simulink library "Feeder2_lib"  (Simulink 8.1)
settings: Solver=ode45  StartTime=0.0  StopTime=10.0  RelTol=1e-3
undefined symbols (not defined in the file): Left, Ts, type, V
libraries: breaker_lib x20, cables_lib x14, transformer_lib x12, Load_lib x8, ssn_lib x7, powerlib x4, fault_lib x2, rtlab x2
settings Model: Creator=re25624  LastModifiedBy=RE25624

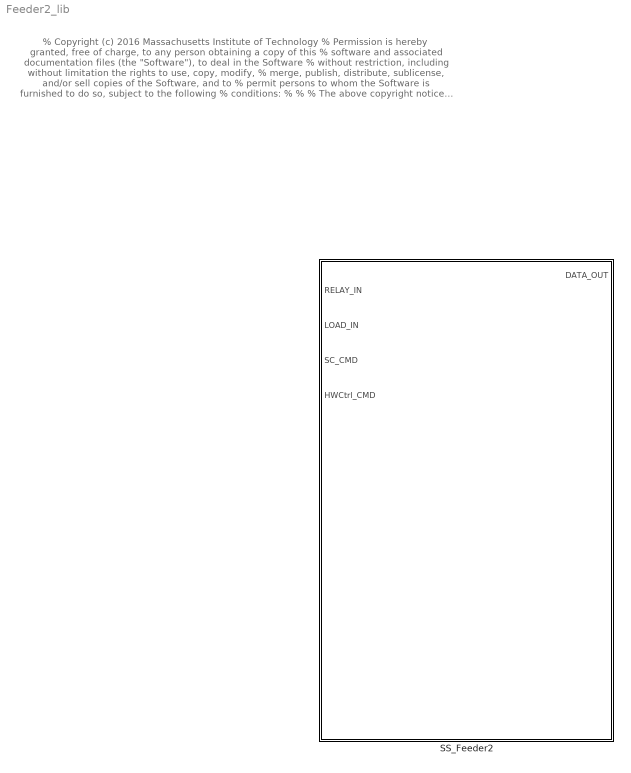
== system Feeder2_lib ==
  note: % Copyright (c) 2016 Massachusetts Institute of Technology
      | % Permission is hereby granted, free of charge, to any person obtaining a copy of this
      | % software and associated documentation files (the "Software"), to deal in the Software
      | % without restriction, including without limitation the rights to use, copy, modify,
      | % merge, publish, distribute, sublicense, and/or sell copies of the Software, and to
      | % permit persons to whom the Software is furnished to do so, subject to the following
      | % conditions:
      | %
      | %
      | % The above copyright notice and this permission notice shall be included in
      | % all copies or substantial portions of the Software.
      | %
      | % THE SOFTWARE IS PROVIDED "AS IS", WITHOUT WARRANTY OF ANY KIND, EXPRESS OR IMPLIED,
      | % INCLUDING BUT NOT LIMITED TO THE WARRANTIES OF MERCHANTABILITY, FITNESS FOR A
      | % PARTICULAR PURPOSE AND NONINFRINGEMENT. IN NO EVENT SHALL THE AUTHORS OR COPYRIGHT
      | % HOLDERS BE LIABLE FOR ANY CLAIM, DAMAGES OR OTHER LIABILITY, WHETHER IN AN ACTION
      | % OF CONTRACT, TORT OR OTHERWISE, ARISING FROM, OUT OF OR IN CONNECTION WITH THE
      | % SOFTWARE OR THE USE OR OTHER DEALINGS IN THE SOFTWARE.
      | %
      | %
      | %%
  SS_Feeder2 : Subsystem

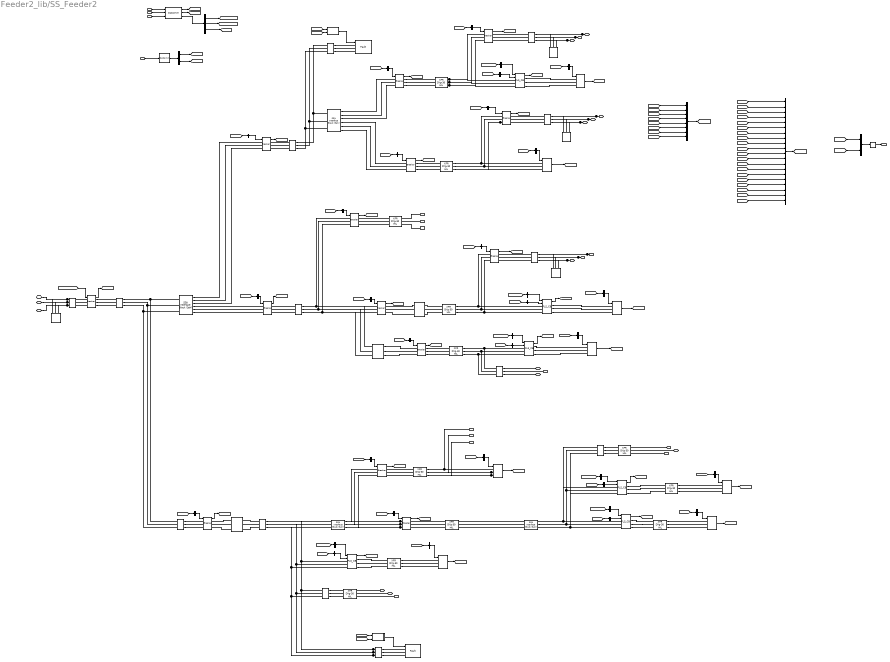
== system Feeder2_lib/SS_Feeder2 ==
  note: BESS SYSTEM
  note: % Copyright (c) 2016 Massachusetts Institute of Technology
      | % Permission is hereby granted, free of charge, to any person obtaining a copy of this
      | % software and associated documentation files (the "Software"), to deal in the Software
      | % without restriction, including without limitation the rights to use, copy, modify,
      | % merge, publish, distribute, sublicense, and/or sell copies of the Software, and to
      | % permit persons to whom the Software is furnished to do so, subject to the following
      | % conditions:
      | %
      | %
      | % The above copyright notice and this permission notice shall be included in
      | % all copies or substantial portions of the Software.
      | %
      | % THE SOFTWARE IS PROVIDED "AS IS", WITHOUT WARRANTY OF ANY KIND, EXPRESS OR IMPLIED,
      | % INCLUDING BUT NOT LIMITED TO THE WARRANTIES OF MERCHANTABILITY, FITNESS FOR A
      | % PARTICULAR PURPOSE AND NONINFRINGEMENT. IN NO EVENT SHALL THE AUTHORS OR COPYRIGHT
      | % HOLDERS BE LIABLE FOR ANY CLAIM, DAMAGES OR OTHER LIABILITY, WHETHER IN AN ACTION
      | % OF CONTRACT, TORT OR OTHERWISE, ARISING FROM, OUT OF OR IN CONNECTION WITH THE
      | % SOFTWARE OR THE USE OR OTHER DEALINGS IN THE SOFTWARE.
      | %
      | %
      | %%
  note: connect to F1
  note: PV SYSTEM
  note: connect to F3
  note: connect to F3
  note: connect to F3
  note: connect to F1
  note: connect to F1
  RELAY_IN : Inport
  LOAD_IN : Inport  Port=2
  SC_CMD : Inport  Port=3
  HWCtrl_CMD : Inport  Port=4
  1000 kVA1 : transformer_lib/XFR DYg-30 HIL  Rating=1000  Vp=13800  Vs=480  Z=4.56  XR=4.49
  1000 kVA2 : transformer_lib/XFR DYg-30 HIL  Rating=1000  Vp=4160  Vs=480  Z=5.56  XR=5.49
  1500 kVA : transformer_lib/XFR DYg-30 HIL  Rating=1500  Vp=4160  Vs=480  Z=5.56  XR=5.51
  2000 kVA2 : transformer_lib/XFR DYg-30 HIL  Rating=2000  Vp=13800  Vs=480  Z=3  XR=5.7
  2000 kVA3 : transformer_lib/XFR DYg-30 HIL  Rating=2000  Vp=13800  Vs=480  Z=3  XR=5.7
  2500 kVA : transformer_lib/XFR DYg-30 HIL  Rating=2500  Vp=13800  Vs=480  Z=5.56  XR=5.52
  2500 kVA1 : transformer_lib/XFR DYg-30 HIL  Rating=2500  Vp=13800  Vs=480  Z=3.56  XR=5.52
  3750 kVA : transformer_lib/XFR DYg-30 HIL  Rating=3750  Vp=13800  Vs=4160  Z=4.75  XR=11.4
  4/0AWG-Mutual : cables_lib/4//0AWG-Mutual  length=10  par_sets=1  ratio=3
  448 kvar inductor at 13.8kV  to cancel kvar produced by the stublines1 : powerlib/Elements/Three-Phase Parallel RLC Load  LConnTagsString=A|B|C  Configuration=Y (grounded)  NominalVoltage=13800  NominalFrequency=60  ActivePower=0  InductivePower=448e3  CapacitivePower=0  Measurements=None  LoadType=constant Z
  500 kVA : transformer_lib/XFR DYg-30 HIL  Rating=500  Vp=13800  Vs=208  Z=5  XR=4.9
  5000 kVA : transformer_lib/XFR DYg-30 HIL  Rating=5000  Vp=13800  Vs=480  Z=3  XR=5.44
  500kcmil-Mutual2 : cables_lib/500kcmil-Mutual  length=10  par_sets=1  ratio=3
  500kcmil-Mutual4 : cables_lib/500kcmil-Mutual  length=10  par_sets=1  ratio=3
  500kcmil-Mutual5 : cables_lib/500kcmil-Mutual  length=1000  par_sets=1  ratio=3
  500kcmil-Mutual8 : cables_lib/500kcmil-Mutual  length=100  par_sets=1  ratio=3
  500kcmil-Mutual9 : cables_lib/500kcmil-Mutual  length=10  par_sets=1  ratio=3
  6 kvar inductor at 480V  to cancel kvar produced by the stublines1 : powerlib/Elements/Three-Phase Parallel RLC Load  LConnTagsString=A|B|C  Configuration=Y (grounded)  NominalVoltage=480  NominalFrequency=60  ActivePower=0  InductivePower=6e3  CapacitivePower=0  Measurements=None  LoadType=constant Z
  6 kvar inductor at 480V  to cancel kvar produced by the stublines2 : powerlib/Elements/Three-Phase Parallel RLC Load  LConnTagsString=A|B|C  Configuration=Y (grounded)  NominalVoltage=480  NominalFrequency=60  ActivePower=0  InductivePower=6e3  CapacitivePower=0  Measurements=None  LoadType=constant Z
  6 kvar inductor at 480V  to cancel kvar produced by the stublines3 : powerlib/Elements/Three-Phase Parallel RLC Load  LConnTagsString=A|B|C  Configuration=Y (grounded)  NominalVoltage=480  NominalFrequency=60  ActivePower=0  InductivePower=6e3  CapacitivePower=0  Measurements=None  LoadType=constant Z
  Bus Creator2 : BusCreator  Inputs=2
  Bus Creator3 : BusCreator  Inputs=8
  Bus Creator5 : BusCreator  Inputs=20
  Bus Selector1 : BusSelector  OutputSignals=F2_CB_4
  Bus Selector10 : BusSelector  OutputSignals=I4
  Bus Selector11 : BusSelector  OutputSignals=F2_CB_11
  Bus Selector12 : BusSelector  OutputSignals=F2_CB_15
  Bus Selector13 : BusSelector  OutputSignals=F2_CB_3
  Bus Selector14 : BusSelector  OutputSignals=F2_CB_14
  Bus Selector15 : BusSelector  OutputSignals=F2_CB_17
  Bus Selector16 : BusSelector  OutputSignals=F2_CB_16
  Bus Selector17 : BusSelector  OutputSignals=F2_CB_13
  Bus Selector18 : BusSelector  OutputSignals=F2_CB_10
  Bus Selector19 : BusSelector  OutputSignals=F2_CB_9
  Bus Selector2 : BusSelector  OutputSignals=F2_CB_2
  Bus Selector20 : BusSelector  OutputSignals=F2_CB_12
  Bus Selector21 : BusSelector  OutputSignals=F2_CB_5
  Bus Selector22 : BusSelector  OutputSignals=F2_CB_7
  Bus Selector23 : BusSelector  OutputSignals=F2_CB_8
  Bus Selector24 : BusSelector  OutputSignals=F2_CB_6
  Bus Selector25 : BusSelector  OutputSignals=F2_CB_1
  Bus Selector26 : BusSelector  OutputSignals=F2_CB_18
  Bus Selector27 : BusSelector  OutputSignals=F2_CB_19
  Bus Selector28 : BusSelector  OutputSignals=fault_cmd,GridStatusCtrl.Grid_F2.Logic_trip
  Bus Selector29 : BusSelector  OutputSignals=HWCtrl.SEL751_LogicTrip.F2.Logic_trip,HWCtrl.SEL2440_FLS,TestSeq
  Bus Selector3 : BusSelector  OutputSignals=P5
  Bus Selector30 : BusSelector  OutputSignals=CB218
  Bus Selector31 : BusSelector  OutputSignals=CB212
  Bus Selector32 : BusSelector  OutputSignals=CB219
  Bus Selector33 : BusSelector  OutputSignals=CB206
  Bus Selector34 : BusSelector  OutputSignals=CB208
  Bus Selector35 : BusSelector  OutputSignals=CB204
  Bus Selector4 : BusSelector  OutputSignals=C4
  Bus Selector5 : BusSelector  OutputSignals=I5
  Bus Selector6 : BusSelector  OutputSignals=P2
  Bus Selector7 : BusSelector  OutputSignals=C3
  Bus Selector8 : BusSelector  OutputSignals=P3
  Bus Selector9 : BusSelector  OutputSignals=I3
  C{1..2,204..206} (5 alike) : cables_lib/500kcmil-Mutual  length=10  par_sets=1  ratio=3
  C201 : cables_lib/4//0AWG-Mutual  length=5500  par_sets=1  ratio=3
  C202 : cables_lib/500kcmil-Mutual  length=2000  par_sets=1  ratio=3
  C203 : cables_lib/500kcmil-Mutual  length=3000  par_sets=1  ratio=3
  Critical_3 : Load_lib/Dynamic_Load  V=480  kVA=1000  PF=0.9  Ts=Ts
  Critical_4 : Load_lib/Dynamic_Load  V=480  kVA=1000  PF=0.9  Ts=Ts
  F2_CB_{1..3,5,7,9..11,13..17} (13 alike) : breaker_lib/Breaker  Ts=Ts  mech_delay=cb_mech_delay
  F2_CB_{4,6,8,12,18..19} (6 alike) : breaker_lib/FLS_CB  Ts=Ts  mech_delay=cb_mech_delay
  F2_PCC : breaker_lib/Breaker  Ts=Ts  mech_delay=cb_mech_delay
  Fault_1 : fault_lib/Fault  FaultResistance=0.1  GroundResistance=1.73  SnubberResistance=1E6
  Fault_5 : fault_lib/Fault  FaultResistance=0.1  GroundResistance=1.73  SnubberResistance=1E6
  Interruptible_3 : Load_lib/Dynamic_Load  V=208  kVA=300  PF=0.9  Ts=Ts
  Interruptible_4 : Load_lib/Dynamic_Load  V=480  kVA=600  PF=0.9  Ts=Ts
  Interruptible_5 : Load_lib/Dynamic_Load  V=480  kVA=400  PF=0.9  Ts=Ts
  Low imp xfr to handle stubline : transformer_lib/XFR DYg-30 HIL  Rating=5000  Vp=13800  Vs=500  Z=0.1  XR=10
  Low imp xfr to handle stubline1 : transformer_lib/XFR DYg-30 HIL  Rating=5000  Vp=4160  Vs=500  Z=0.1  XR=10
  Memory : Memory
  OpComm1 : rtlab/OpComm  nbport=3  groupe_acq=1  subsys_rate=0  st=0  Synchronization=on  Interpolation=on  Threshold=1.0  Missed_Data=off  Sim_Time=off  Samples=off  dynSigOut=off  from_console=0  warning_done=off  writeOpCommFile=off  Offset=off
  OpComm2 : rtlab/OpComm  nbport=1  groupe_acq=1  subsys_rate=0  st=0  Synchronization=on  Interpolation=on  Threshold=1.0  Missed_Data=off  Sim_Time=off  Samples=off  dynSigOut=off  from_console=1  warning_done=off  writeOpCommFile=off  Offset=off
  Priority_2 : Load_lib/Dynamic_Load  V=480  kVA=1000  PF=0.9  Ts=Ts
  Priority_3 : Load_lib/Dynamic_Load  V=480  kVA=1000  PF=0.9  Ts=Ts
  Priority_5 : Load_lib/Dynamic_Load  V=480  kVA=700  PF=0.9  Ts=Ts
  SSN Interface Block (3ph){1,3,5,9..10} (5 alike) : ssn_lib/SSN Interface Block (3ph)  nb_phase=3  nb_port=2  p1_type=V-type(Left)  p2_type=V-type (Right)  p3_type=V-type(Left)  p4_type=V-type(Left)  p5_type=V-type(Left)  p6_type=V-type(Left)  p7_type=V-type(Left)  p8_type=V-type(Left)  p9_type=V-type(Left)  p10_type=V-type(Left)  p11_type=V-type(Left)  p12_type=V-type(Left)  p13_type=V-type(Left)  p14_type=V-type(Left)  p15_type=V-type(Left)  p16_type=V-type(Left)  I_port_shunt_resistance=1e9
  SSN Interface Block (3ph)2 : ssn_lib/SSN Interface Block (3ph)  nb_phase=3  nb_port=3  p1_type=V-type(Left)  p2_type=V-type (Right)  p3_type=V-type (Right)  p4_type=V-type(Left)  p5_type=V-type(Left)  p6_type=V-type(Left)  p7_type=V-type(Left)  p8_type=V-type(Left)  p9_type=V-type(Left)  p10_type=V-type(Left)  p11_type=V-type(Left)  p12_type=V-type(Left)  p13_type=V-type(Left)  p14_type=V-type(Left)  p15_type=V-type(Left)  p16_type=V-type(Left)  I_port_shunt_resistance=1e9
  SSN Interface Block (3ph)4 : ssn_lib/SSN Interface Block (3ph)  nb_phase=3  nb_port=3  p1_type=V-type(Left)  p2_type=V-type (Right)  p3_type=V-type (Right)  p4_type=V-type(Left)  p5_type=V-type(Left)  p6_type=V-type(Left)  p7_type=V-type(Left)  p8_type=V-type(Left)  p9_type=V-type(Left)  p10_type=V-type(Left)  p11_type=V-type(Left)  p12_type=V-type(Left)  p13_type=V-type(Left)  p14_type=V-type(Left)  p15_type=V-type(Left)  p16_type=V-type(Left)  I_port_shunt_resistance=1e9
  fault_signal : Subsystem
  fault_signal1 : Subsystem
  A_CB_13 : PMIOPort  Port=1  Side=Right
  B_CB_13 : PMIOPort  Port=2  Side=Right
  C_CB_13 : PMIOPort  Port=3  Side=Right
  A_CB_17 : PMIOPort  Port=4  Side=Right
  B_CB_17 : PMIOPort  Port=5  Side=Right
  C_CB_17 : PMIOPort  Port=6  Side=Right
  A_CB_16 : PMIOPort  Port=7  Side=Right
  B_CB_16 : PMIOPort  Port=8  Side=Right
  C_CB_16 : PMIOPort  Port=9  Side=Right
  A_CB_9 : PMIOPort  Port=10  Side=Right
  B_CB_9 : PMIOPort  Port=11  Side=Right
  C_CB_9 : PMIOPort  Port=12  Side=Right
  A_CB_7 : PMIOPort  Port=13  Side=Right
  B_CB_7 : PMIOPort  Port=14  Side=Right
  C_CB_7 : PMIOPort  Port=15  Side=Right
  A_CB_1 : PMIOPort  Port=16  Side=Right
  B_CB_1 : PMIOPort  Port=17  Side=Right
  C_CB_1 : PMIOPort  Port=18  Side=Right
  PCC_A : PMIOPort  Port=19  Side=Left
  PCC_B : PMIOPort  Port=20  Side=Left
  PCC_C : PMIOPort  Port=21  Side=Left
  A_PV : PMIOPort  Port=22  Side=Left
  B_PV : PMIOPort  Port=23  Side=Left
  C_PV : PMIOPort  Port=24  Side=Left
  A_BESS : PMIOPort  Port=25  Side=Left
  B_BESS : PMIOPort  Port=26  Side=Left
  C_BESS : PMIOPort  Port=27  Side=Left
  DATA_OUT : Outport
  wires:
  fault_signal1/1(o) -> Fault_1/1
  [fault_cmd] -> fault_signal1/2(fault_sc)
  [TestSeq] -> fault_signal1/1(fault_ts)
  fault_signal/1(o) -> Fault_5/1
  [fault_cmd] -> fault_signal/2(fault_sc)
  [TestSeq] -> fault_signal/1(fault_ts)
  Bus Selector29/3 -> [TestSeq]  "<TestSeq>"
  Bus Selector28/2 -> [feeder_cb]  "<Logic_trip>"
  Bus Selector29/2 -> [SEL_2440_FLS]  "<SEL2440_FLS>"
  F2_CB_18/1 -> [F2_CB_18]
  Bus Selector35/1 -> F2_CB_4/1  "<CB204>"
  [SEL_2440_FLS] -> Bus Selector35/1
  Bus Selector34/1 -> F2_CB_8/1  "<CB208>"
  [SEL_2440_FLS] -> Bus Selector34/1
  Bus Selector33/1 -> F2_CB_6/1  "<CB206>"
  [SEL_2440_FLS] -> Bus Selector33/1
  Bus Selector32/1 -> F2_CB_19/1  "<CB219>"
  [SEL_2440_FLS] -> Bus Selector32/1
  Bus Selector31/1 -> F2_CB_12/1  "<CB212>"
  [SEL_2440_FLS] -> Bus Selector31/1
  Bus Selector30/1 -> F2_CB_18/1  "<CB218>"
  [SEL_2440_FLS] -> Bus Selector30/1
  OpComm1/3 -> Bus Selector29/1
  Bus Selector29/1 -> [SEL751_F2_LogicTrip]  "<Logic_trip>"
  HWCtrl_CMD/1 -> OpComm1/3
  [SEL751_F2_LogicTrip] -> F2_PCC/1
  [LOAD_DATA] -> Bus Creator2/2  "LOAD_DATA"
  [CB_DATA] -> Bus Creator2/1  "CB_DATA"
  Bus Creator5/1 -> [CB_DATA]
  Bus Creator2/1 -> Memory/1
  Bus Selector28/1 -> [fault_cmd]  "<fault_cmd>"
  OpComm2/1 -> Bus Selector28/1
  Memory/1 -> DATA_OUT/1
  SC_CMD/1 -> OpComm2/1
  Bus Selector27/1 -> F2_CB_19/2  "<F2_CB_19>"
  [RELAY_IN] -> Bus Selector27/1
  F2_CB_19/1 -> [F2_CB_19]
  [F2_CB_19] -> Bus Creator5/19  "F2_CB_19"
  [F2_CB_18] -> Bus Creator5/18  "F2_CB_18"
  Bus Selector26/1 -> F2_CB_18/2  "<F2_CB_18>"
  [RELAY_IN] -> Bus Selector26/1
  Bus Selector1/1 -> F2_CB_4/2  "<F2_CB_4>"
  [RELAY_IN] -> Bus Selector1/1
  F2_CB_4/1 -> [F2_CB_4]
  [F2_PCC] -> Bus Creator5/20  "F2_PCC"
  F2_PCC/1 -> [F2_PCC]
  F2_CB_16/1 -> [F2_CB_16]
  F2_CB_12/1 -> [F2_CB_12]
  Bus Selector15/1 -> F2_CB_17/1  "<F2_CB_17>"
  [F2_CB_17] -> Bus Creator5/17  "F2_CB_17"
  Bus Selector23/1 -> F2_CB_8/2  "<F2_CB_8>"
  Bus Selector24/1 -> F2_CB_6/2  "<F2_CB_6>"
  Bus Selector22/1 -> F2_CB_7/1  "<F2_CB_7>"
  Bus Selector21/1 -> F2_CB_5/1  "<F2_CB_5>"
  Bus Selector25/1 -> F2_CB_1/1  "<F2_CB_1>"
  Bus Selector12/1 -> F2_CB_15/1  "<F2_CB_15>"
  Bus Selector16/1 -> F2_CB_16/1  "<F2_CB_16>"
  Bus Selector14/1 -> F2_CB_14/1  "<F2_CB_14>"
  Bus Selector20/1 -> F2_CB_12/2  "<F2_CB_12>"
  Bus Selector17/1 -> F2_CB_13/1  "<F2_CB_13>"
  Bus Selector19/1 -> F2_CB_9/1  "<F2_CB_9>"
  Bus Selector18/1 -> F2_CB_10/1  "<F2_CB_10>"
  Bus Selector11/1 -> F2_CB_11/1  "<F2_CB_11>"
  Bus Selector2/1 -> F2_CB_2/1  "<F2_CB_2>"
  [RELAY_IN] -> Bus Selector25/1
  [RELAY_IN] -> Bus Selector24/1
  [RELAY_IN] -> Bus Selector23/1
  [RELAY_IN] -> Bus Selector22/1
  [RELAY_IN] -> Bus Selector21/1
  [RELAY_IN] -> Bus Selector20/1
  [RELAY_IN] -> Bus Selector19/1
  [RELAY_IN] -> Bus Selector18/1
  [RELAY_IN] -> Bus Selector17/1
  [RELAY_IN] -> Bus Selector16/1
  [RELAY_IN] -> Bus Selector15/1
  [RELAY_IN] -> Bus Selector14/1
  [RELAY_IN] -> Bus Selector12/1
  [RELAY_IN] -> Bus Selector11/1
  [RELAY_IN] -> Bus Selector2/1
  [RELAY_IN] -> Bus Selector13/1
  Bus Selector13/1 -> F2_CB_3/1  "<F2_CB_3>"
  OpComm1/2 -> [RELAY_IN]
  RELAY_IN/1 -> OpComm1/2
  [F2_CB_16] -> Bus Creator5/16  "F2_CB_16"
  [F2_CB_15] -> Bus Creator5/15  "F2_CB_15"
  [F2_CB_13] -> Bus Creator5/13  "F2_CB_13"
  [F2_CB_10] -> Bus Creator5/10  "F2_CB_10"
  [F2_CB_12] -> Bus Creator5/12  "F2_CB_12"
  [F2_CB_8] -> Bus Creator5/8  "F2_CB_8"
  [F2_CB_5] -> Bus Creator5/5  "F2_CB_5"
  [F2_CB_14] -> Bus Creator5/14  "F2_CB_14"
  [F2_CB_11] -> Bus Creator5/11  "F2_CB_11"
  [F2_CB_7] -> Bus Creator5/7  "F2_CB_7"
  [F2_CB_9] -> Bus Creator5/9  "F2_CB_9"
  [F2_CB_4] -> Bus Creator5/4  "F2_CB_4"
  [F2_CB_6] -> Bus Creator5/6  "F2_CB_6"
  [F2_CB_3] -> Bus Creator5/3  "F2_CB_3"
  [F2_CB_2] -> Bus Creator5/2  "F2_CB_2"
  [F2_CB_1] -> Bus Creator5/1  "F2_CB_1"
  F2_CB_13/1 -> [F2_CB_13]
  F2_CB_10/1 -> [F2_CB_10]
  F2_CB_14/1 -> [F2_CB_14]
  F2_CB_17/1 -> [F2_CB_17]
  F2_CB_15/1 -> [F2_CB_15]
  F2_CB_11/1 -> [F2_CB_11]
  F2_CB_3/1 -> [F2_CB_3]
  F2_CB_9/1 -> [F2_CB_9]
  F2_CB_8/1 -> [F2_CB_8]
  F2_CB_5/1 -> [F2_CB_5]
  F2_CB_7/1 -> [F2_CB_7]
  F2_CB_6/1 -> [F2_CB_6]
  F2_CB_1/1 -> [F2_CB_1]
  F2_CB_2/1 -> [F2_CB_2]
  [LOAD_P5] -> Bus Creator3/8  "F2_P5"
  [LOAD_P3] -> Bus Creator3/7  "F2_P3"
  [LOAD_I3] -> Bus Creator3/3  "F2_I3"
  [LOAD_C4] -> Bus Creator3/2  "F2_C4"
  [LOAD_I5] -> Bus Creator3/5  "F2_I5"
  [LOAD_P2] -> Bus Creator3/6  "F2_P2"
  [LOAD_I4] -> Bus Creator3/4  "F2_I4"
  Bus Creator3/1 -> [LOAD_DATA]  "LOAD"
  [LOAD_C3] -> Bus Creator3/1  "F2_C3"
  Interruptible_4/1 -> [LOAD_I4]
  Priority_3/1 -> [LOAD_P3]
  Interruptible_3/1 -> [LOAD_I3]
  Critical_3/1 -> [LOAD_C3]
  Priority_2/1 -> [LOAD_P2]
  Interruptible_5/1 -> [LOAD_I5]
  Priority_5/1 -> [LOAD_P5]
  Critical_4/1 -> [LOAD_C4]
  Bus Selector9/1 -> Interruptible_3/1  "<I3>"
  Bus Selector10/1 -> Interruptible_4/1  "<I4>"
  Bus Selector8/1 -> Priority_3/1  "<P3>"
  Bus Selector7/1 -> Critical_3/1  "<C3>"
  Bus Selector6/1 -> Priority_2/1  "<P2>"
  Bus Selector5/1 -> Interruptible_5/1  "<I5>"
  Bus Selector4/1 -> Critical_4/1  "<C4>"
  Bus Selector3/1 -> Priority_5/1  "<P5>"
  [LOAD_IN] -> Bus Selector10/1
  [LOAD_IN] -> Bus Selector9/1
  [LOAD_IN] -> Bus Selector8/1
  [LOAD_IN] -> Bus Selector7/1
  [LOAD_IN] -> Bus Selector6/1
  [LOAD_IN] -> Bus Selector5/1
  [LOAD_IN] -> Bus Selector4/1
  [LOAD_IN] -> Bus Selector3/1
  OpComm1/1 -> [LOAD_IN]
  LOAD_IN/1 -> OpComm1/1
  connections:
  C2/RConn1 -- Low imp xfr to handle stubline/LConn1
  C2/RConn3 -- Low imp xfr to handle stubline/LConn3
  C2/RConn2 -- Low imp xfr to handle stubline/LConn2
  C1/RConn1 -- Low imp xfr to handle stubline1/LConn1
  C1/RConn3 -- Low imp xfr to handle stubline1/LConn3
  C1/RConn2 -- Low imp xfr to handle stubline1/LConn2
  F2_CB_8/LConn1 -- SSN Interface Block (3ph)1/RConn1 -- C1/LConn1 -- F2_CB_4/LConn1
  B_CB_7/RConn1 -- Low imp xfr to handle stubline1/RConn2
  A_CB_7/RConn1 -- Low imp xfr to handle stubline1/RConn1
  C_CB_7/RConn1 -- Low imp xfr to handle stubline1/RConn3
  C_CB_1/RConn1 -- Low imp xfr to handle stubline/RConn3
  B_CB_1/RConn1 -- Low imp xfr to handle stubline/RConn2
  A_CB_1/RConn1 -- Low imp xfr to handle stubline/RConn1
  F2_CB_4/LConn2 -- C1/LConn2 -- SSN Interface Block (3ph)1/RConn2 -- F2_CB_8/LConn2
  F2_CB_8/LConn3 -- SSN Interface Block (3ph)1/RConn3 -- C1/LConn3 -- F2_CB_4/LConn3
  500kcmil-Mutual2/LConn2 -- C2/LConn2 -- C201/RConn2 -- SSN Interface Block (3ph)5/LConn2 -- F2_CB_6/LConn2
  500kcmil-Mutual2/LConn1 -- C2/LConn1 -- C201/RConn1 -- SSN Interface Block (3ph)5/LConn1 -- F2_CB_6/LConn1
  500kcmil-Mutual2/LConn3 -- C2/LConn3 -- C201/RConn3 -- SSN Interface Block (3ph)5/LConn3 -- F2_CB_6/LConn3
  B_PV/RConn1 -- 5000 kVA/RConn2
  C_PV/RConn1 -- 5000 kVA/RConn3
  A_PV/RConn1 -- 5000 kVA/RConn1
  500kcmil-Mutual2/RConn1 -- Fault_1/LConn1
  500kcmil-Mutual2/RConn3 -- Fault_1/LConn3
  500kcmil-Mutual2/RConn2 -- Fault_1/LConn2
  500kcmil-Mutual9/RConn1 -- Fault_5/LConn1
  500kcmil-Mutual9/RConn3 -- Fault_5/LConn3
  500kcmil-Mutual9/RConn2 -- Fault_5/LConn2
  SSN Interface Block (3ph)1/LConn1 -- 3750 kVA/RConn1
  SSN Interface Block (3ph)1/LConn2 -- 3750 kVA/RConn2
  SSN Interface Block (3ph)1/LConn3 -- 3750 kVA/RConn3
  F2_CB_7/LConn3 -- F2_CB_5/LConn3 -- SSN Interface Block (3ph)5/RConn3
  F2_CB_7/LConn1 -- F2_CB_5/LConn1 -- SSN Interface Block (3ph)5/RConn1
  F2_CB_7/LConn2 -- F2_CB_5/LConn2 -- SSN Interface Block (3ph)5/RConn2
  C201/LConn3 -- SSN Interface Block (3ph)10/RConn3
  C201/LConn1 -- SSN Interface Block (3ph)10/RConn1
  C201/LConn2 -- SSN Interface Block (3ph)10/RConn2
  SSN Interface Block (3ph)10/LConn1 -- F2_CB_1/RConn1
  SSN Interface Block (3ph)10/LConn2 -- F2_CB_1/RConn2
  SSN Interface Block (3ph)10/LConn3 -- F2_CB_1/RConn3
  4/0AWG-Mutual/RConn3 -- F2_CB_1/LConn3
  4/0AWG-Mutual/RConn1 -- F2_CB_1/LConn1
  4/0AWG-Mutual/RConn2 -- F2_CB_1/LConn2
  500kcmil-Mutual5/LConn3 -- 448 kvar inductor at 13.8kV  to cancel kvar produced by the stublines1/LConn3 -- PCC_C/RConn1
  500kcmil-Mutual5/LConn1 -- 448 kvar inductor at 13.8kV  to cancel kvar produced by the stublines1/LConn1 -- PCC_A/RConn1
  500kcmil-Mutual5/LConn2 -- 448 kvar inductor at 13.8kV  to cancel kvar produced by the stublines1/LConn2 -- PCC_B/RConn1
  F2_CB_18/RConn1 -- Priority_5/LConn1
  F2_PCC/LConn1 -- 500kcmil-Mutual5/RConn1
  F2_PCC/LConn2 -- 500kcmil-Mutual5/RConn2
  F2_PCC/LConn3 -- 500kcmil-Mutual5/RConn3
  F2_PCC/RConn3 -- 500kcmil-Mutual8/LConn3
  F2_PCC/RConn2 -- 500kcmil-Mutual8/LConn2
  F2_PCC/RConn1 -- 500kcmil-Mutual8/LConn1
  500kcmil-Mutual4/RConn2 -- B_CB_9/RConn1
  500kcmil-Mutual4/RConn3 -- C_CB_9/RConn1
  500kcmil-Mutual4/RConn1 -- A_CB_9/RConn1
  500 kVA/RConn1 -- Interruptible_3/LConn1
  500 kVA/RConn3 -- Interruptible_3/LConn3
  500 kVA/RConn2 -- Interruptible_3/LConn2
  1000 kVA2/RConn3 -- Interruptible_4/LConn3
  1000 kVA2/RConn2 -- Interruptible_4/LConn2
  1000 kVA2/RConn1 -- Interruptible_4/LConn1
  Critical_3/LConn2 -- B_BESS/RConn1 -- 2500 kVA/RConn2
  Critical_3/LConn3 -- C_BESS/RConn1 -- 2500 kVA/RConn3
  A_BESS/RConn1 -- Critical_3/LConn1 -- 2500 kVA/RConn1
  SSN Interface Block (3ph)2/RConn4 -- F2_CB_14/LConn1
  SSN Interface Block (3ph)2/RConn5 -- F2_CB_14/LConn2
  SSN Interface Block (3ph)2/RConn6 -- F2_CB_14/LConn3
  SSN Interface Block (3ph)2/RConn3 -- F2_CB_15/LConn3
  SSN Interface Block (3ph)2/RConn2 -- F2_CB_15/LConn2
  SSN Interface Block (3ph)2/RConn1 -- F2_CB_15/LConn1
  C202/LConn3 -- F2_CB_2/RConn3
  C202/LConn1 -- F2_CB_2/RConn1
  C202/LConn2 -- F2_CB_2/RConn2
  SSN Interface Block (3ph)4/RConn4 -- F2_CB_2/LConn1
  SSN Interface Block (3ph)4/RConn6 -- F2_CB_2/LConn3
  SSN Interface Block (3ph)4/RConn5 -- F2_CB_2/LConn2
  F2_CB_4/RConn1 -- 1500 kVA/LConn1
  F2_CB_4/RConn2 -- 1500 kVA/LConn2
  F2_CB_4/RConn3 -- 1500 kVA/LConn3
  1500 kVA/RConn1 -- Priority_3/LConn1
  1500 kVA/RConn2 -- Priority_3/LConn2
  1500 kVA/RConn3 -- Priority_3/LConn3
  A_CB_13/RConn1 -- 6 kvar inductor at 480V  to cancel kvar produced by the stublines3/LConn1 -- C206/RConn1
  B_CB_13/RConn1 -- 6 kvar inductor at 480V  to cancel kvar produced by the stublines3/LConn2 -- C206/RConn2
  C_CB_13/RConn1 -- 6 kvar inductor at 480V  to cancel kvar produced by the stublines3/LConn3 -- C206/RConn3
  C206/LConn1 -- F2_CB_13/RConn1
  C206/LConn2 -- F2_CB_13/RConn2
  C206/LConn3 -- F2_CB_13/RConn3
  A_CB_17/RConn1 -- 6 kvar inductor at 480V  to cancel kvar produced by the stublines2/LConn1 -- C205/RConn1
  B_CB_17/RConn1 -- 6 kvar inductor at 480V  to cancel kvar produced by the stublines2/LConn2 -- C205/RConn2
  C_CB_17/RConn1 -- 6 kvar inductor at 480V  to cancel kvar produced by the stublines2/LConn3 -- C205/RConn3
  C205/LConn2 -- F2_CB_17/RConn2
  C205/LConn1 -- F2_CB_17/RConn1
  C205/LConn3 -- F2_CB_17/RConn3
  A_CB_16/RConn1 -- 6 kvar inductor at 480V  to cancel kvar produced by the stublines1/LConn1 -- C204/RConn1
  B_CB_16/RConn1 -- 6 kvar inductor at 480V  to cancel kvar produced by the stublines1/LConn2 -- C204/RConn2
  C_CB_16/RConn1 -- 6 kvar inductor at 480V  to cancel kvar produced by the stublines1/LConn3 -- C204/RConn3
  C204/LConn2 -- F2_CB_16/RConn2
  C204/LConn1 -- F2_CB_16/RConn1
  C204/LConn3 -- F2_CB_16/RConn3
  SSN Interface Block (3ph)3/RConn1 -- F2_CB_9/LConn1
  SSN Interface Block (3ph)3/RConn3 -- F2_CB_9/LConn3
  SSN Interface Block (3ph)3/RConn2 -- F2_CB_9/LConn2
  F2_CB_19/RConn3 -- Priority_2/LConn3
  F2_CB_19/RConn2 -- Priority_2/LConn2
  F2_CB_19/RConn1 -- Priority_2/LConn1
  F2_CB_18/RConn3 -- Priority_5/LConn3
  F2_CB_18/RConn2 -- Priority_5/LConn2
  F2_CB_19/LConn3 -- 500kcmil-Mutual4/LConn3 -- 2500 kVA1/RConn3
  F2_CB_19/LConn1 -- 500kcmil-Mutual4/LConn1 -- 2500 kVA1/RConn1
  F2_CB_9/RConn2 -- 2500 kVA1/LConn2
  SSN Interface Block (3ph)4/LConn3 -- 500kcmil-Mutual8/RConn3 -- 4/0AWG-Mutual/LConn3
  500kcmil-Mutual8/RConn2 -- 4/0AWG-Mutual/LConn2 -- SSN Interface Block (3ph)4/LConn2
  F2_CB_6/RConn1 -- 500 kVA/LConn1
  F2_CB_15/RConn2 -- 2000 kVA3/LConn2
  F2_CB_11/LConn1 -- C202/RConn1 -- F2_CB_10/LConn1 -- SSN Interface Block (3ph)3/LConn1
  3750 kVA/LConn1 -- F2_CB_7/RConn1
  3750 kVA/LConn2 -- F2_CB_7/RConn2
  2000 kVA2/RConn2 -- F2_CB_17/LConn2 -- Critical_4/LConn2
  5000 kVA/LConn3 -- F2_CB_11/RConn3
  C203/LConn2 -- F2_CB_3/RConn2
  F2_CB_19/LConn2 -- 500kcmil-Mutual4/LConn2 -- 2500 kVA1/RConn2
  F2_CB_9/RConn1 -- 2500 kVA1/LConn1
  F2_CB_15/RConn3 -- 2000 kVA3/LConn3
  5000 kVA/LConn1 -- F2_CB_11/RConn1
  F2_CB_17/LConn3 -- 2000 kVA2/RConn3 -- Critical_4/LConn3
  F2_CB_15/RConn1 -- 2000 kVA3/LConn1
  F2_CB_14/RConn1 -- 2000 kVA2/LConn1
  SSN Interface Block (3ph)9/LConn1 -- F2_CB_10/RConn1
  2000 kVA3/RConn1 -- F2_CB_18/LConn1 -- F2_CB_16/LConn1
  2500 kVA/LConn2 -- F2_CB_5/RConn2
  2500 kVA/LConn3 -- F2_CB_5/RConn3
  2500 kVA/LConn1 -- F2_CB_5/RConn1
  SSN Interface Block (3ph)9/LConn2 -- F2_CB_10/RConn2
  C203/LConn1 -- F2_CB_3/RConn1
  C203/LConn3 -- F2_CB_3/RConn3
  3750 kVA/LConn3 -- F2_CB_7/RConn3
  500kcmil-Mutual8/RConn1 -- 4/0AWG-Mutual/LConn1 -- SSN Interface Block (3ph)4/LConn1
  F2_CB_11/LConn2 -- C202/RConn2 -- SSN Interface Block (3ph)3/LConn2 -- F2_CB_10/LConn2
  2000 kVA2/RConn1 -- F2_CB_17/LConn1 -- Critical_4/LConn1
  5000 kVA/LConn2 -- F2_CB_11/RConn2
  2000 kVA3/RConn3 -- F2_CB_18/LConn3 -- F2_CB_16/LConn3
  F2_CB_6/RConn3 -- 500 kVA/LConn3
  F2_CB_11/LConn3 -- C202/RConn3 -- F2_CB_10/LConn3 -- SSN Interface Block (3ph)3/LConn3
  F2_CB_9/RConn3 -- 2500 kVA1/LConn3
  SSN Interface Block (3ph)9/LConn3 -- F2_CB_10/RConn3
  F2_CB_6/RConn2 -- 500 kVA/LConn2
  F2_CB_14/RConn2 -- 2000 kVA2/LConn2
  2000 kVA3/RConn2 -- F2_CB_18/LConn2 -- F2_CB_16/LConn2
  F2_CB_14/RConn3 -- 2000 kVA2/LConn3
  SSN Interface Block (3ph)4/RConn2 -- F2_CB_3/LConn2
  SSN Interface Block (3ph)4/RConn1 -- F2_CB_3/LConn1
  SSN Interface Block (3ph)4/RConn3 -- F2_CB_3/LConn3
  F2_CB_8/RConn2 -- 1000 kVA2/LConn2
  F2_CB_8/RConn1 -- 1000 kVA2/LConn1
  F2_CB_8/RConn3 -- 1000 kVA2/LConn3
  1000 kVA1/LConn2 -- SSN Interface Block (3ph)9/RConn2
  1000 kVA1/LConn3 -- SSN Interface Block (3ph)9/RConn3
  1000 kVA1/LConn1 -- SSN Interface Block (3ph)9/RConn1
  F2_CB_12/RConn1 -- Interruptible_5/LConn1
  F2_CB_12/RConn2 -- Interruptible_5/LConn2
  F2_CB_12/RConn3 -- Interruptible_5/LConn3
  1000 kVA1/RConn3 -- F2_CB_12/LConn3 -- F2_CB_13/LConn3
  1000 kVA1/RConn2 -- F2_CB_12/LConn2 -- F2_CB_13/LConn2
  1000 kVA1/RConn1 -- F2_CB_12/LConn1 -- F2_CB_13/LConn1
  500kcmil-Mutual9/LConn3 -- C203/RConn3 -- SSN Interface Block (3ph)2/LConn3
  500kcmil-Mutual9/LConn2 -- C203/RConn2 -- SSN Interface Block (3ph)2/LConn2
  500kcmil-Mutual9/LConn1 -- C203/RConn1 -- SSN Interface Block (3ph)2/LConn1

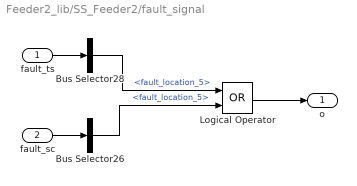
== system Feeder2_lib/SS_Feeder2/fault_signal ==
  fault_ts : Inport
  fault_sc : Inport  Port=2
  Bus Selector26 : BusSelector  OutputSignals=fault_location_5
  Bus Selector28 : BusSelector  OutputSignals=fault_location_5
  Logical Operator : Logic  Operator=OR  AllPortsSameDT=off  OutDataTypeStr=boolean
  o : Outport
  wires:
  Bus Selector28/1 -> Logical Operator/1  "<fault_location_5>"
  Logical Operator/1 -> o/1
  fault_ts/1 -> Bus Selector28/1
  Bus Selector26/1 -> Logical Operator/2  "<fault_location_5>"
  fault_sc/1 -> Bus Selector26/1

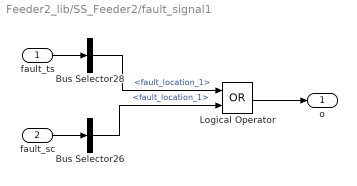
== system Feeder2_lib/SS_Feeder2/fault_signal1 ==
  fault_ts : Inport
  fault_sc : Inport  Port=2
  Bus Selector26 : BusSelector  OutputSignals=fault_location_1
  Bus Selector28 : BusSelector  OutputSignals=fault_location_1
  Logical Operator : Logic  Operator=OR  AllPortsSameDT=off  OutDataTypeStr=boolean
  o : Outport
  wires:
  Bus Selector28/1 -> Logical Operator/1  "<fault_location_1>"
  Logical Operator/1 -> o/1
  fault_ts/1 -> Bus Selector28/1
  Bus Selector26/1 -> Logical Operator/2  "<fault_location_1>"
  fault_sc/1 -> Bus Selector26/1
